simulink model "SVPWM"  (R2024b)
settings: Solver=VariableStepAuto  StartTime=0.0  StopTime=10.0  RelTol=1e-3
settings Model: Creator=misaka10039  LastModifiedBy=misaka10039

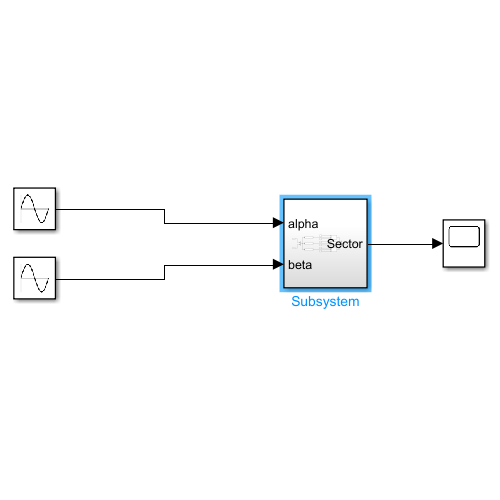
[thumbnail: Simulink's stored preview of the top-level diagram]
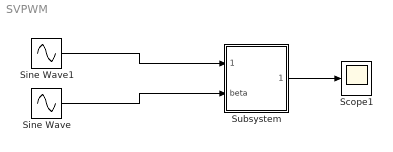
== system SVPWM ==
  Scope1 : Scope
  Sine Wave : Sin  Amplitude=200  Frequency=100*pi  SampleTime=0
  Sine Wave1 : Sin  Amplitude=200  Frequency=100*pi  Phase=pi/2  SampleTime=0
  Subsystem : Subsystem
  wires:
  Sine Wave/1 -> Subsystem/2(beta)
  Sine Wave1/1 -> Subsystem/1(alpha)
  Subsystem/1(Sector) -> Scope1/1

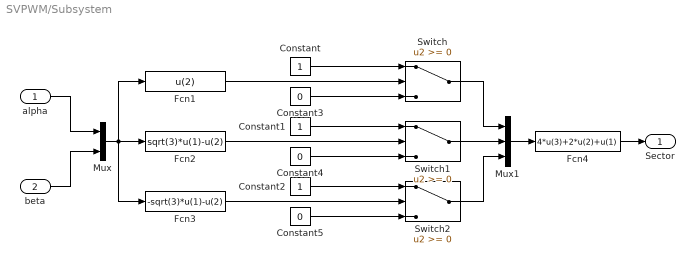
== system SVPWM/Subsystem ==
  alpha : Inport
  beta : Inport  Port=2
  Constant : Constant
  Constant1 : Constant
  Constant2 : Constant
  Constant3 : Constant  Value=0
  Constant4 : Constant  Value=0
  Constant5 : Constant  Value=0
  Fcn1 : Fcn  Expr=u(2)
  Fcn2 : Fcn  Expr=sqrt(3)*u(1)-u(2)
  Fcn3 : Fcn  Expr=-sqrt(3)*u(1)-u(2)
  Fcn4 : Fcn  Expr=4*u(3)+2*u(2)+u(1)
  Mux : Mux  Inputs=2
  Mux1 : Mux  Inputs=3
  Switch : Switch  SaturateOnIntegerOverflow=off  InputSameDT=off
  Switch1 : Switch  SaturateOnIntegerOverflow=off  InputSameDT=off
  Switch2 : Switch  SaturateOnIntegerOverflow=off  InputSameDT=off
  Sector : Outport
  wires:
  Switch1/1 -> Mux1/2
  Constant1/1 -> Switch1/1
  Constant5/1 -> Switch2/3
  Mux/1 -> Fcn3/1, Fcn1/1, Fcn2/1
  beta/1 -> Mux/2
  Constant3/1 -> Switch/3
  alpha/1 -> Mux/1
  Constant4/1 -> Switch1/3
  Constant/1 -> Switch/1
  Fcn1/1 -> Switch/2
  Fcn3/1 -> Switch2/2
  Switch2/1 -> Mux1/3
  Constant2/1 -> Switch2/1
  Switch/1 -> Mux1/1
  Mux1/1 -> Fcn4/1
  Fcn2/1 -> Switch1/2
  Fcn4/1 -> Sector/1
